simulink model "QA_test"  (R2018a)
settings: Solver=ode113  StartTime=0.0  StopTime=t(end)  RelTol=1e-6
values from neighbouring files (symbols this model uses):
  K = 1.5e9    (= 1500000000)    [plot_TLM_error_map.m]    (also in plot_TLM_interpolation_error_map.m)
  L = 100    [plot_TLM_error_map.m]    (also in plot_TLM_interpolation_error_map.m)
  rA = 12e-3    (= 0.012)    [plot_TLM_error_map.m]    (also in plot_TLM_interpolation_error_map.m)
  rB = lambdaA*rA    [plot_TLM_error_map.m]    (also in plot_TLM_interpolation_error_map.m)
libraries: usask_segmented_TLM_lib x1
settings Model: Creator=tkw954  LastModifiedBy=tkw954
settings DataIOCC: ReturnWorkspaceOutputs=on  OutputOption=SpecifiedOutputTimes  OutputTimes=t

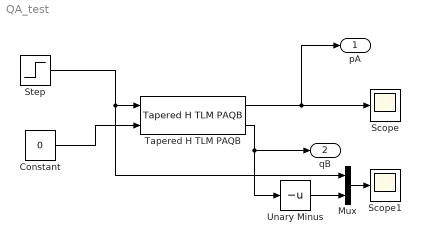
== system QA_test ==
  Constant : Constant  Value=0
  Mux : Mux  Inputs=2
  Scope : Scope
  Scope1 : Scope
  Step : Step  Time=0  SampleTime=0
  Tapered H TLM PAQB : usask_segmented_TLM_lib/Tapered H TLM PAQB  D_A=rA*2  D_B=rB*2  L=L  K=K  nu=nu  rho=rho
  Unary Minus : UnaryMinus
  pA : Outport
  qB : Outport  Port=2
  wires:
  Constant/1 -> Tapered H TLM PAQB/2
  Step/1 -> Tapered H TLM PAQB/1, Mux/1
  Tapered H TLM PAQB/1 -> pA/1, Scope/1
  Mux/1 -> Scope1/1
  Tapered H TLM PAQB/2 -> qB/1, Unary Minus/1
  Unary Minus/1 -> Mux/2
